simulink model "st_transient_ODE1"  (R2025b)
settings: Solver=VariableStepAuto  StartTime=0.0  StopTime=10.0  RelTol=1e-3
values from neighbouring files (symbols this model uses):
  A_oins = 0.6*pi*r3    [st_transient_parameters.m]
  mcp_RP1 = m_RP1*cp_RP1 + m_wall*cp_al    (= 61.4260182409)    [st_transient_parameters.m]
  R_ins = 0    [st_transient_parameters.m]
  T_RP1_i = 290    [st_transient_parameters.m]
settings Model: Creator=aryan  LastModifiedBy=aryan

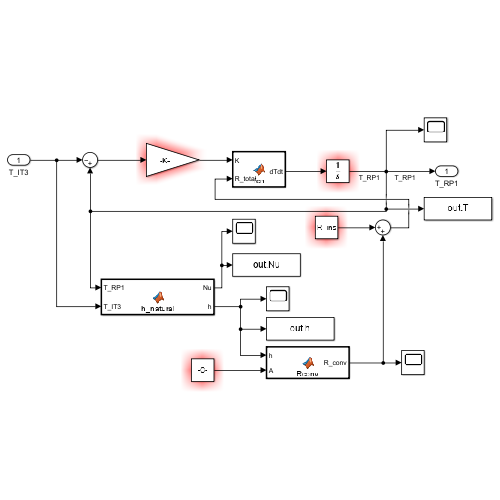
[thumbnail: Simulink's stored preview of the top-level diagram]
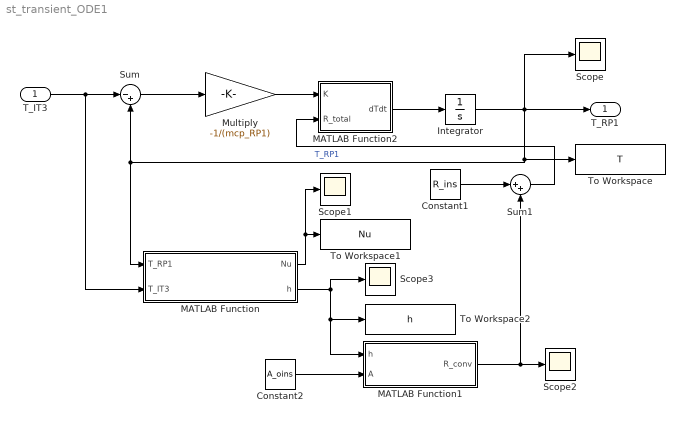
== system st_transient_ODE1 ==
  T_IT3 : Inport
  Constant1 : Constant  Value=R_ins
  Constant2 : Constant  Value=A_oins
  Integrator : Integrator  InitialCondition=T_RP1_i
  MATLAB Function : MATLAB Function  TreatAsAtomicUnit=on
  MATLAB Function1 : MATLAB Function  TreatAsAtomicUnit=on
  MATLAB Function2 : MATLAB Function  TreatAsAtomicUnit=on
  Multiply : Gain  Gain=-1/(mcp_RP1)
  Scope{,1..3} (4 alike) : Scope
      Scope settings: ActiveDisplayYMinimum=260.25246238308375  ActiveDisplayYMaximum=321.33069422822069
      Scope1 settings: ActiveDisplayYMinimum=-1  ActiveDisplayYMaximum=1
      Scope2 settings: ActiveDisplayYMinimum=-31.29088337884123  ActiveDisplayYMaximum=45.896592661263512  DataLoggingVariableName=ScopeData2
      Scope3 settings: ActiveDisplayYMinimum=-1.453026566225704  ActiveDisplayYMaximum=14.066469860499284  DataLoggingVariableName=ScopeData3
  Sum : Sum  Inputs=|-+
  Sum1 : Sum  Inputs=|++
  To Workspace : ToWorkspace  VariableName=T  SaveFormat=Timeseries  SampleTime=-1
  To Workspace1 : ToWorkspace  VariableName=Nu  SaveFormat=Timeseries  SampleTime=-1
  To Workspace2 : ToWorkspace  VariableName=h  SaveFormat=Timeseries  SampleTime=-1
  T_RP1 : Outport
  wires:
  Integrator/1 -> T_RP1/1, MATLAB Function/1(T_RP1), Sum/2, To Workspace/1, Scope/1  "T_RP1"
  Sum1/1 -> MATLAB Function2/2(R_total)
  MATLAB Function2/1(dTdt) -> Integrator/1
  MATLAB Function/2(h) -> Scope3/1, To Workspace2/1, MATLAB Function1/1(h)
  Multiply/1 -> MATLAB Function2/1(K)
  Sum/1 -> Multiply/1
  Constant2/1 -> MATLAB Function1/2(A)
  MATLAB Function/1(Nu) -> To Workspace1/1, Scope1/1
  Constant1/1 -> Sum1/1
  MATLAB Function1/1(R_conv) -> Sum1/2, Scope2/1
  T_IT3/1 -> MATLAB Function/2(T_IT3), Sum/1

== matlab function st_transient_ODE1/MATLAB Function1 ==
  data: h input; R_conv output; A input
function R_conv = Rconv(h, A)

    R_conv = 1/(h*A);

== matlab function st_transient_ODE1/MATLAB Function ==
  data: Nu output; h output; T_RP1 input; T_IT3 input
function [Nu, h] = h_natural(T_RP1, T_IT3)
    coder.extrinsic('getNusselt_natural')
    Nu = 0;
    h = 0;

    geo = 'vertical_plate';
    rho = 1.225;    % {kg/m^3}              T = 290 K, P within [0.5, 40] MPa
    mu = 0.001;     % {Pa*s}                T = 293 K
    k = 0.135;      % {W/m*K}
    cp = 1005;      % {J/kg*K}
    L = 0.127;      % {m}
    D = 0;          % {m} not needed for case: 'vertical_plate'
    
    % T_film = (T_IT3 + T_i)/2
    [Nu, h] = getNusselt_natural(geo, rho, mu, k, cp, L, D, T_RP1, T_IT3);

== matlab function st_transient_ODE1/MATLAB Function2 ==
  data: K input; R_total input; dTdt output
function dTdt = fcn(K, R_total)
    
    dTdt = K/R_total;
